simulink model "Dynamic_model_of_Dc_Machine_Qudus"  (R2023a)
settings: Solver=VariableStepAuto  StartTime=0.0  StopTime=0.1  RelTol=1e-3
settings Model: Creator=QUDUS  LastModifiedBy=QUDUS

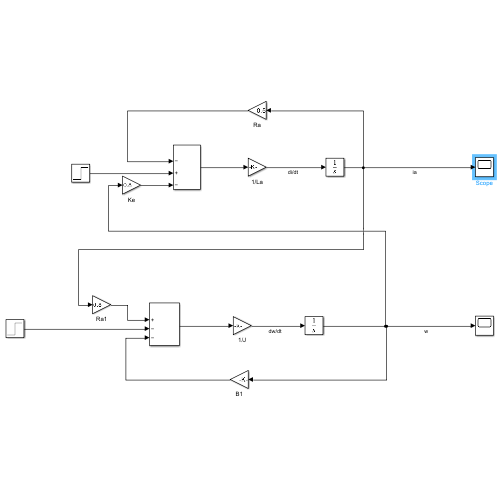
[thumbnail: Simulink's stored preview of the top-level diagram]
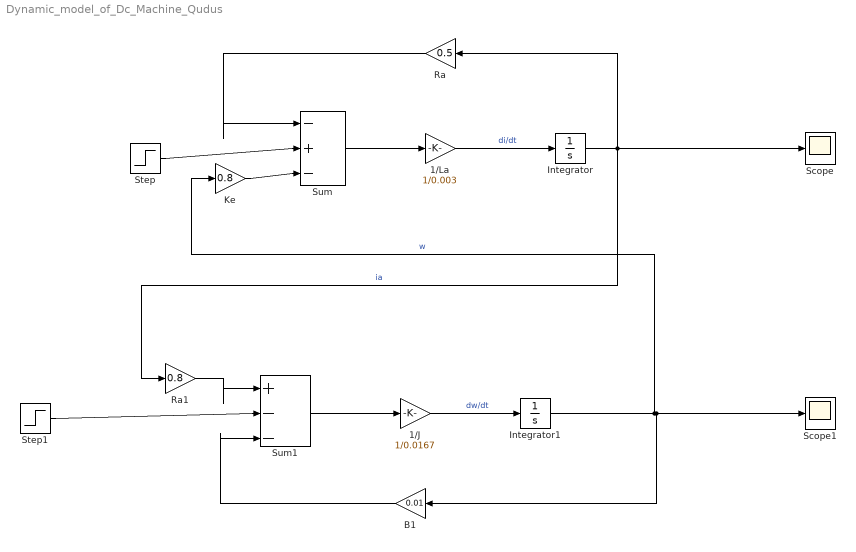
== system Dynamic_model_of_Dc_Machine_Qudus ==
  1/J : Gain  Gain=1/0.0167
  1/La : Gain  Gain=1/0.003
  B1 : Gain  Gain=0.01
  Integrator : Integrator
  Integrator1 : Integrator
  Ke : Gain  Gain=0.8
  Ra : Gain  Gain=0.5
  Ra1 : Gain  Gain=0.8
  Scope : Scope
  Scope1 : Scope
  Step : Step  Time=0  After=220  SampleTime=0
  Step1 : Step  Time=0  After=100  SampleTime=0
  Sum : Sum  Inputs=|-+-
  Sum1 : Sum  Inputs=|+--
  wires:
  Step/1 -> Sum/2
  Ke/1 -> Sum/3
  Ra/1 -> Sum/1
  Sum/1 -> 1/La/1
  1/La/1 -> Integrator/1  "di/dt"
  Integrator/1 -> Ra1/1, Scope/1, Ra/1  "ia"
  1/J/1 -> Integrator1/1  "dw/dt"
  Step1/1 -> Sum1/2
  Sum1/1 -> 1/J/1
  Ra1/1 -> Sum1/1
  B1/1 -> Sum1/3
  Integrator1/1 -> Ke/1, B1/1, Scope1/1  "w"
